simulink model "pmsmParameter"  (R2018a)
settings: Solver=VariableStepAuto  StartTime=0.0  StopTime=0.5  MaxStep=1e-6  RelTol=1e-6
libraries: powerlib x48, simulink x1
settings Model: Creator=R-YDL  LastModifiedBy=R-YDL

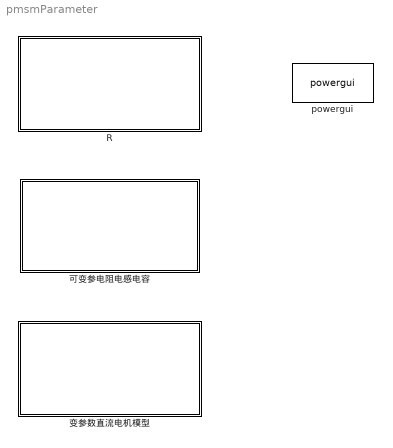
== system pmsmParameter ==
  R : Subsystem  mask{Vset=10, R=2}
      mask prompts: Vset "电压设置"; R "电阻Omega"
  powergui : powerlib/powergui  Priority=1  SimulationMode=Continuous  SampleTime=50e-6  frequency=60  Iterations=50  frequencyindice=0  Pbase=100e6  ErrMax=1e-4  UnitsV=kV  UnitsW=MW  buscounter=0  FunctionMessages=off  echomessages=off  EnableUseOfTLC=off  CurrentSourceSwitches=off  DisableSnubberDevices=off  DisableRonSwitches=off  DisableVfSwitches=off  DisplayEquations=off  SolverType=Tustin/Backward Euler (TBE)  Interpol=off  ExternalGateDelay=off  methode=off  Ts=100  x0status=blocks  SPID=on  SwTol=0  HookPort=off  RestoreLinks=warning  ResistiveCurrentMeasurement=off  Frange=[0:2:500]  Ylog=off  Xlog=on  ShowGrid=off  save=off  variable=ZData  structure=0  ZoomFFT=off  StartTime=0.0  cycles=1  DisplayStyle=1  fundamental=60  FreqAxis=off  MaxFrequency=1000  frequencyindicesteady=1  RmsSteady=1  display=off
  变参数直流电机模型 : Subsystem  mask{Vset=10, R=2, L=1e-2, C=1e-3, J=10, KE=1.8, KT=17.2}
      mask prompts: Vset "电源电压"; R "电枢电阻"; L "电枢电感"; C "电枢电容"; J "转动惯量（kg.m^3）"; KE "反电动势系数"; KT "电磁转矩系数（N.m/A）"
  可变参电阻电感电容 : Subsystem  mask{Vset=10, R=5, L=1e-2, C=1e-3}
      mask prompts: Vset "电压设置"; R "电阻Omega"; L "电感(H)"; C "电容(F)"

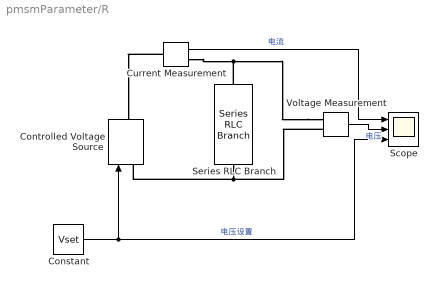
== system pmsmParameter/R ==
  Constant : Constant  Value=Vset
  Controlled Voltage Source : powerlib/Electrical Sources/Controlled Voltage Source  Initialize=on  Source_Type=AC  Amplitude=0  Phase=0  Frequency=0  Measurements=None
  Current Measurement : powerlib/Measurements/Current Measurement  PhasorSimulation=off  OutputType=Complex  PSBequivalent=0
  Scope : Scope  NumInputPorts=3
  Series RLC Branch : powerlib/Elements/Series RLC Branch  LConnTagsString=__new0  RConnTagsString=__new0  BranchType=R  Resistance=R  Inductance=1e-3  SetiL0=off  InitialCurrent=0  Capacitance=1e-6  Setx0=off  InitialVoltage=0  Measurements=None
  Voltage Measurement : powerlib/Measurements/Voltage Measurement  PhasorSimulation=off  OutputType=Complex  PSBequivalent=0
  wires:
  Current Measurement/1 -> Scope/1  "电流"
  Constant/1 -> Controlled Voltage Source/1, Scope/3  "电压设置"
  Voltage Measurement/1 -> Scope/2  "电压"
  connections:
  Voltage Measurement/LConn1 -- Series RLC Branch/LConn1 -- Current Measurement/RConn1
  Controlled Voltage Source/LConn1 -- Voltage Measurement/LConn2 -- Series RLC Branch/RConn1
  Current Measurement/LConn1 -- Controlled Voltage Source/RConn1

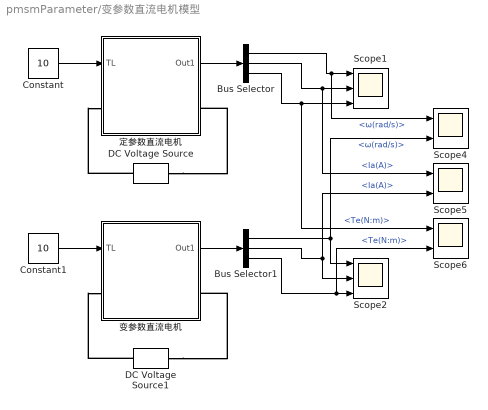
== system pmsmParameter/变参数直流电机模型 ==
  Bus Selector : BusSelector  OutputSignals=ω(rad/s),Ia(A),Te(N:m)
  Bus Selector1 : BusSelector  OutputSignals=ω(rad/s),Ia(A),Te(N:m)
  Constant : Constant  Value=10
  Constant1 : Constant  Value=10
  DC Voltage Source : powerlib/Electrical Sources/DC Voltage Source  Amplitude=12  Measurements=None
  DC Voltage Source1 : powerlib/Electrical Sources/DC Voltage Source  Amplitude=12  Measurements=None
  Scope1 : Scope  NumInputPorts=3
  Scope2 : Scope  NumInputPorts=3
  Scope4 : Scope  NumInputPorts=2
  Scope5 : Scope  NumInputPorts=2
  Scope6 : Scope  NumInputPorts=2
  变参数直流电机 : Subsystem
  定参数直流电机 : Subsystem
  wires:
  Constant/1 -> 定参数直流电机/1(TL)
  定参数直流电机/1(Out1) -> Bus Selector/1
  Bus Selector/1 -> Scope4/1, Scope1/1  "<ω(rad/s)>"
  Bus Selector/2 -> Scope5/1, Scope1/2  "<Ia(A)>"
  Bus Selector/3 -> Scope6/1, Scope1/3  "<Te(N:m)>"
  变参数直流电机/1(Out1) -> Bus Selector1/1
  Bus Selector1/3 -> Scope6/2, Scope2/3  "<Te(N:m)>"
  Bus Selector1/1 -> Scope2/1, Scope4/2  "<ω(rad/s)>"
  Constant1/1 -> 变参数直流电机/1(TL)
  Bus Selector1/2 -> Scope5/2, Scope2/2  "<Ia(A)>"
  connections:
  DC Voltage Source/RConn1 -- 定参数直流电机/LConn1
  DC Voltage Source/LConn1 -- 定参数直流电机/RConn1
  DC Voltage Source1/RConn1 -- 变参数直流电机/LConn1
  DC Voltage Source1/LConn1 -- 变参数直流电机/RConn1

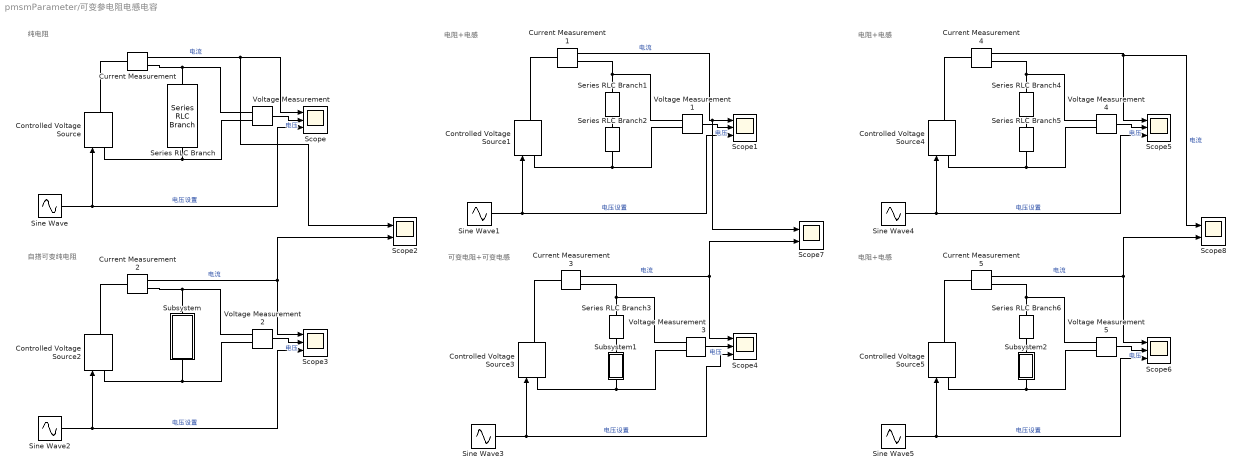
== system pmsmParameter/可变参电阻电感电容 ==
  note: 电阻+电感
  note: 纯电阻
  note: 自搭可变纯电阻
  note: 可变电阻+可变电感
  note: 电阻+电感
  note: 电阻+电感
  Controlled Voltage Source{,1..5} (6 alike) : powerlib/Electrical Sources/Controlled Voltage Source  Initialize=on  Source_Type=AC  Amplitude=0  Phase=0  Frequency=0  Measurements=None
  Current Measurement{,1..5} (6 alike) : powerlib/Measurements/Current Measurement  PhasorSimulation=off  OutputType=Complex  PSBequivalent=0
  Scope{,1,3..6} (6 alike) : Scope  NumInputPorts=3
  Scope2 : Scope  NumInputPorts=2
  Scope7 : Scope  NumInputPorts=2
  Scope8 : Scope  NumInputPorts=2
  Series RLC Branch{,1,3..4,6} (5 alike) : powerlib/Elements/Series RLC Branch  LConnTagsString=__new0  RConnTagsString=__new0  BranchType=R  Resistance=R  Inductance=1e-3  SetiL0=off  InitialCurrent=0  Capacitance=1e-6  Setx0=off  InitialVoltage=0  Measurements=None
  Series RLC Branch2 : powerlib/Elements/Series RLC Branch  LConnTagsString=__new0  RConnTagsString=__new0  BranchType=L  Resistance=R  Inductance=L  SetiL0=off  InitialCurrent=0  Capacitance=1e-6  Setx0=off  InitialVoltage=0  Measurements=None
  Series RLC Branch5 : powerlib/Elements/Series RLC Branch  LConnTagsString=__new0  RConnTagsString=__new0  BranchType=C  Resistance=R  Inductance=L  SetiL0=off  InitialCurrent=0  Capacitance=C  Setx0=off  InitialVoltage=0  Measurements=None
  Sine Wave{,1..5} (6 alike) : Sin  Amplitude=Vset  Frequency=50*2*pi  SampleTime=0
  Subsystem : Subsystem
  Subsystem1 : Subsystem
  Subsystem2 : Subsystem
  Voltage Measurement{,1..5} (6 alike) : powerlib/Measurements/Voltage Measurement  PhasorSimulation=off  OutputType=Complex  PSBequivalent=0
  wires:
  Current Measurement/1 -> Scope2/1, Scope/1  "电流"
  Sine Wave/1 -> Controlled Voltage Source/1, Scope/3  "电压设置"
  Voltage Measurement/1 -> Scope/2  "电压"
  Sine Wave1/1 -> Controlled Voltage Source1/1, Scope1/3  "电压设置"
  Voltage Measurement1/1 -> Scope1/2  "电压"
  Current Measurement1/1 -> Scope7/1, Scope1/1  "电流"
  Sine Wave2/1 -> Controlled Voltage Source2/1, Scope3/3  "电压设置"
  Voltage Measurement2/1 -> Scope3/2  "电压"
  Current Measurement2/1 -> Scope2/2, Scope3/1  "电流"
  Sine Wave3/1 -> Controlled Voltage Source3/1, Scope4/3  "电压设置"
  Voltage Measurement3/1 -> Scope4/2  "电压"
  Current Measurement3/1 -> Scope7/2, Scope4/1  "电流"
  Sine Wave4/1 -> Controlled Voltage Source4/1, Scope5/3  "电压设置"
  Voltage Measurement4/1 -> Scope5/2  "电压"
  Current Measurement4/1 -> Scope8/1, Scope5/1  "电流"
  Current Measurement5/1 -> Scope8/2, Scope6/1  "电流"
  Sine Wave5/1 -> Controlled Voltage Source5/1, Scope6/3  "电压设置"
  Voltage Measurement5/1 -> Scope6/2  "电压"
  connections:
  Current Measurement/RConn1 -- Voltage Measurement/LConn1 -- Series RLC Branch/LConn1
  Series RLC Branch/RConn1 -- Controlled Voltage Source/LConn1 -- Voltage Measurement/LConn2
  Current Measurement/LConn1 -- Controlled Voltage Source/RConn1
  Voltage Measurement1/LConn2 -- Series RLC Branch2/RConn1 -- Controlled Voltage Source1/LConn1
  Voltage Measurement1/LConn1 -- Series RLC Branch1/LConn1 -- Current Measurement1/RConn1
  Current Measurement1/LConn1 -- Controlled Voltage Source1/RConn1
  Voltage Measurement2/LConn2 -- Subsystem/RConn1 -- Controlled Voltage Source2/LConn1
  Voltage Measurement2/LConn1 -- Subsystem/LConn1 -- Current Measurement2/RConn1
  Current Measurement2/LConn1 -- Controlled Voltage Source2/RConn1
  Series RLC Branch2/LConn1 -- Series RLC Branch1/RConn1
  Current Measurement3/RConn1 -- Series RLC Branch3/LConn1 -- Voltage Measurement3/LConn1
  Controlled Voltage Source3/LConn1 -- Subsystem1/RConn1 -- Voltage Measurement3/LConn2
  Subsystem1/LConn1 -- Series RLC Branch3/RConn1
  Current Measurement3/LConn1 -- Controlled Voltage Source3/RConn1
  Current Measurement4/RConn1 -- Voltage Measurement4/LConn1 -- Series RLC Branch4/LConn1
  Controlled Voltage Source4/LConn1 -- Voltage Measurement4/LConn2 -- Series RLC Branch5/RConn1
  Series RLC Branch5/LConn1 -- Series RLC Branch4/RConn1
  Current Measurement4/LConn1 -- Controlled Voltage Source4/RConn1
  Current Measurement5/RConn1 -- Voltage Measurement5/LConn1 -- Series RLC Branch6/LConn1
  Controlled Voltage Source5/LConn1 -- Subsystem2/RConn1 -- Voltage Measurement5/LConn2
  Subsystem2/LConn1 -- Series RLC Branch6/RConn1
  Current Measurement5/LConn1 -- Controlled Voltage Source5/RConn1

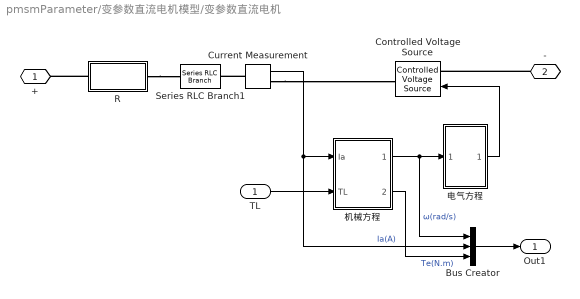
== system pmsmParameter/变参数直流电机模型/变参数直流电机 ==
  TL : Inport
  Bus Creator : BusCreator  Inputs=3
  Controlled Voltage Source : powerlib/Electrical Sources/Controlled Voltage Source  Initialize=on  Source_Type=AC  Amplitude=0  Phase=0  Frequency=0  Measurements=None
  Current Measurement : powerlib/Measurements/Current Measurement  PhasorSimulation=off  OutputType=Complex  PSBequivalent=0
  R : Subsystem
  Series RLC Branch1 : powerlib/Elements/Series RLC Branch  LConnTagsString=__new0  RConnTagsString=__new0  BranchType=L  Resistance=1  Inductance=L  SetiL0=off  InitialCurrent=0  Capacitance=1e-6  Setx0=off  InitialVoltage=0  Measurements=None
  机械方程 : Subsystem
  电气方程 : Subsystem
  + : PMIOPort  Side=Left
  - : PMIOPort  Port=2  Side=Right
  Out1 : Outport
  wires:
  Current Measurement/1 -> Bus Creator/2, 机械方程/1(Ia)  "Ia(A)"
  TL/1 -> 机械方程/2(TL)
  电气方程/1(Out1) -> Controlled Voltage Source/1
  Bus Creator/1 -> Out1/1
  机械方程/1(ω(rad/s)) -> Bus Creator/1, 电气方程/1(In1)  "ω(rad/s)"
  机械方程/2(Te(Nm)) -> Bus Creator/3  "Te(N.m)"
  connections:
  R/LConn1 -- +/RConn1
  R/RConn1 -- Series RLC Branch1/LConn1
  Current Measurement/LConn1 -- Series RLC Branch1/RConn1
  Current Measurement/RConn1 -- Controlled Voltage Source/RConn1
  -/RConn1 -- Controlled Voltage Source/LConn1

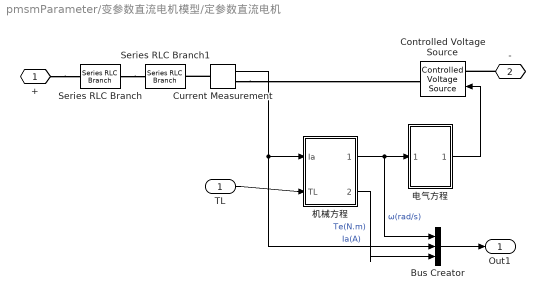
== system pmsmParameter/变参数直流电机模型/定参数直流电机 ==
  TL : Inport
  Bus Creator : BusCreator  Inputs=3
  Controlled Voltage Source : powerlib/Electrical Sources/Controlled Voltage Source  Initialize=on  Source_Type=AC  Amplitude=0  Phase=0  Frequency=0  Measurements=None
  Current Measurement : powerlib/Measurements/Current Measurement  PhasorSimulation=off  OutputType=Complex  PSBequivalent=0
  Series RLC Branch : powerlib/Elements/Series RLC Branch  LConnTagsString=__new0  RConnTagsString=__new0  BranchType=R  Resistance=R  Inductance=1e-3  SetiL0=off  InitialCurrent=0  Capacitance=1e-6  Setx0=off  InitialVoltage=0  Measurements=None
  Series RLC Branch1 : powerlib/Elements/Series RLC Branch  LConnTagsString=__new0  RConnTagsString=__new0  BranchType=L  Resistance=1  Inductance=L  SetiL0=off  InitialCurrent=0  Capacitance=1e-6  Setx0=off  InitialVoltage=0  Measurements=None
  机械方程 : Subsystem
  电气方程 : Subsystem
  + : PMIOPort  Side=Left
  - : PMIOPort  Port=2  Side=Right
  Out1 : Outport
  wires:
  Current Measurement/1 -> Bus Creator/2, 机械方程/1(Ia)  "Ia(A)"
  TL/1 -> 机械方程/2(TL)
  电气方程/1(Out1) -> Controlled Voltage Source/1
  Bus Creator/1 -> Out1/1
  机械方程/1(ω(rad/s)) -> Bus Creator/1, 电气方程/1(In1)  "ω(rad/s)"
  机械方程/2(Te(Nm)) -> Bus Creator/3  "Te(N.m)"
  connections:
  +/RConn1 -- Series RLC Branch/LConn1
  Series RLC Branch/RConn1 -- Series RLC Branch1/LConn1
  Current Measurement/LConn1 -- Series RLC Branch1/RConn1
  Current Measurement/RConn1 -- Controlled Voltage Source/RConn1
  -/RConn1 -- Controlled Voltage Source/LConn1

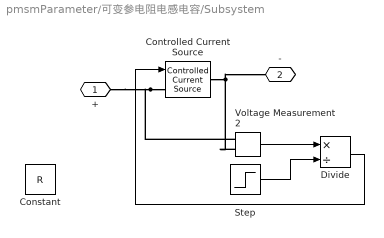
== system pmsmParameter/可变参电阻电感电容/Subsystem ==
  Constant : Constant  Value=R
  Controlled Current Source : powerlib/Electrical Sources/Controlled Current Source  Initialize=on  Source_Type=AC  Amplitude=0  Phase=0  Frequency=0  Measurements=None
  Divide : Product  Inputs=*/
  Step : Step  Time=0.1  Before=R  After=R*2  SampleTime=0
  Voltage Measurement2 : powerlib/Measurements/Voltage Measurement  PhasorSimulation=off  OutputType=Complex  PSBequivalent=0
  + : PMIOPort  Side=Left
  - : PMIOPort  Port=2  Side=Right
  wires:
  Voltage Measurement2/1 -> Divide/1
  Divide/1 -> Controlled Current Source/1
  Step/1 -> Divide/2
  connections:
  Controlled Current Source/LConn1 -- +/RConn1 -- Voltage Measurement2/LConn1
  Controlled Current Source/RConn1 -- -/RConn1 -- Voltage Measurement2/LConn2

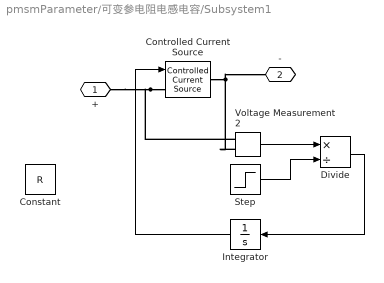
== system pmsmParameter/可变参电阻电感电容/Subsystem1 ==
  Constant : Constant  Value=R
  Controlled Current Source : powerlib/Electrical Sources/Controlled Current Source  Initialize=on  Source_Type=AC  Amplitude=0  Phase=0  Frequency=0  Measurements=None
  Divide : Product  Inputs=*/
  Integrator : Integrator
  Step : Step  Time=0.1  Before=L  After=L*2  SampleTime=0
  Voltage Measurement2 : powerlib/Measurements/Voltage Measurement  PhasorSimulation=off  OutputType=Complex  PSBequivalent=0
  + : PMIOPort  Side=Left
  - : PMIOPort  Port=2  Side=Right
  wires:
  Voltage Measurement2/1 -> Divide/1
  Divide/1 -> Integrator/1
  Step/1 -> Divide/2
  Integrator/1 -> Controlled Current Source/1
  connections:
  Controlled Current Source/LConn1 -- +/RConn1 -- Voltage Measurement2/LConn1
  Controlled Current Source/RConn1 -- -/RConn1 -- Voltage Measurement2/LConn2

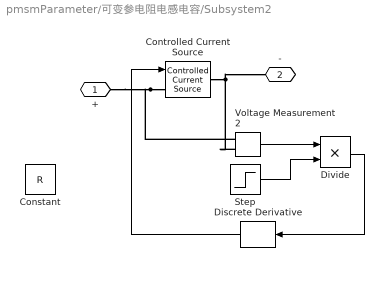
== system pmsmParameter/可变参电阻电感电容/Subsystem2 ==
  Constant : Constant  Value=R
  Controlled Current Source : powerlib/Electrical Sources/Controlled Current Source  Initialize=on  Source_Type=AC  Amplitude=0  Phase=0  Frequency=0  Measurements=None
  Discrete Derivative : simulink/Discrete/Discrete Derivative  gainval=1.0  ICPrevScaledInput=0.0  OutMin=[]  OutMax=[]  OutDataType=fixdt(1, 16)  OutScaling=2^-10  DoSatur=off
  Divide : Product  Inputs=**
  Step : Step  Time=0.1  Before=C  After=C*2  SampleTime=0
  Voltage Measurement2 : powerlib/Measurements/Voltage Measurement  PhasorSimulation=off  OutputType=Complex  PSBequivalent=0
  + : PMIOPort  Side=Left
  - : PMIOPort  Port=2  Side=Right
  wires:
  Voltage Measurement2/1 -> Divide/1
  Divide/1 -> Discrete Derivative/1
  Step/1 -> Divide/2
  Discrete Derivative/1 -> Controlled Current Source/1
  connections:
  Controlled Current Source/LConn1 -- +/RConn1 -- Voltage Measurement2/LConn1
  Controlled Current Source/RConn1 -- -/RConn1 -- Voltage Measurement2/LConn2

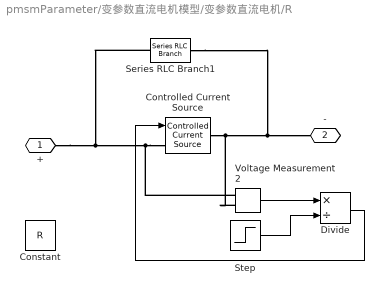
== system pmsmParameter/变参数直流电机模型/变参数直流电机/R ==
  Constant : Constant  Value=R
  Controlled Current Source : powerlib/Electrical Sources/Controlled Current Source  Initialize=on  Source_Type=AC  Amplitude=0  Phase=0  Frequency=0  Measurements=None
  Divide : Product  Inputs=*/
  Series RLC Branch1 : powerlib/Elements/Series RLC Branch  LConnTagsString=__new0  RConnTagsString=__new0  BranchType=R  Resistance=1e5  Inductance=L  SetiL0=off  InitialCurrent=0  Capacitance=1e-6  Setx0=off  InitialVoltage=0  Measurements=None
  Step : Step  Time=0.2  Before=R  After=R*2  SampleTime=0
  Voltage Measurement2 : powerlib/Measurements/Voltage Measurement  PhasorSimulation=off  OutputType=Complex  PSBequivalent=0
  + : PMIOPort  Side=Left
  - : PMIOPort  Port=2  Side=Right
  wires:
  Voltage Measurement2/1 -> Divide/1
  Divide/1 -> Controlled Current Source/1
  Step/1 -> Divide/2
  connections:
  Controlled Current Source/LConn1 -- Series RLC Branch1/LConn1 -- +/RConn1 -- Voltage Measurement2/LConn1
  Controlled Current Source/RConn1 -- Series RLC Branch1/RConn1 -- -/RConn1 -- Voltage Measurement2/LConn2

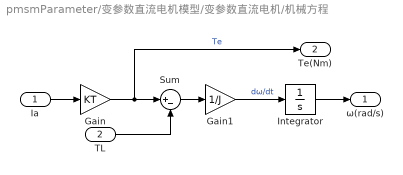
== system pmsmParameter/变参数直流电机模型/变参数直流电机/机械方程 ==
  Ia : Inport
  TL : Inport  Port=2
  Gain : Gain  Gain=KT
  Gain1 : Gain  Gain=1/J
  Integrator : Integrator
  Sum : Sum  Inputs=|+-
  ω(rad/s) : Outport
  Te(Nm) : Outport  Port=2
  wires:
  Gain1/1 -> Integrator/1  "dω/dt"
  Sum/1 -> Gain1/1
  TL/1 -> Sum/2
  Gain/1 -> Te(Nm)/1, Sum/1  "Te"
  Integrator/1 -> ω(rad/s)/1
  Ia/1 -> Gain/1

== system pmsmParameter/变参数直流电机模型/变参数直流电机/电气方程 ==
  In1 : Inport
  V/rpm : Gain  Gain=KE
  rad/s2V/rpm1 : Gain  Gain=30/pi
  Out1 : Outport
  wires:
  rad/s2V/rpm1/1 -> V/rpm/1
  V/rpm/1 -> Out1/1
  In1/1 -> rad/s2V/rpm1/1

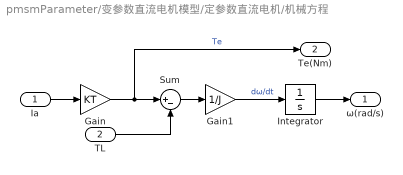
== system pmsmParameter/变参数直流电机模型/定参数直流电机/机械方程 ==
  Ia : Inport
  TL : Inport  Port=2
  Gain : Gain  Gain=KT
  Gain1 : Gain  Gain=1/J
  Integrator : Integrator
  Sum : Sum  Inputs=|+-
  ω(rad/s) : Outport
  Te(Nm) : Outport  Port=2
  wires:
  Gain1/1 -> Integrator/1  "dω/dt"
  Sum/1 -> Gain1/1
  TL/1 -> Sum/2
  Gain/1 -> Te(Nm)/1, Sum/1  "Te"
  Integrator/1 -> ω(rad/s)/1
  Ia/1 -> Gain/1

== system pmsmParameter/变参数直流电机模型/定参数直流电机/电气方程 ==
  In1 : Inport
  V/rpm : Gain  Gain=KE
  rad/s2V/rpm1 : Gain  Gain=30/pi
  Out1 : Outport
  wires:
  rad/s2V/rpm1/1 -> V/rpm/1
  V/rpm/1 -> Out1/1
  In1/1 -> rad/s2V/rpm1/1
